simulink model "Led_Switch_Charts"  (R2018b)
settings: Solver=VariableStepAuto  StartTime=0.0  StopTime=10.0  RelTol=1e-3
settings Model: Creator=mostafa  LastModifiedBy=mostafa

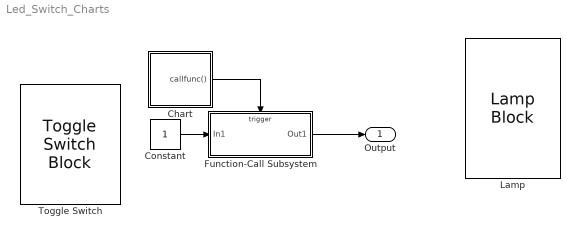
== system Led_Switch_Charts ==
  Chart : Stateflow chart  TreatAsAtomicUnit=on
  Constant : Constant
  Function-Call Subsystem : Subsystem  TreatAsAtomicUnit=on
  Lamp : LampBlock  WebBlockId=14
  Toggle Switch : ToggleSwitchBlock  WebBlockId=11
      settings: Values={{'Off', 'On'}, [0 1]}
  "Output " : Outport
  wires:
  Function-Call Subsystem/1(Out1) -> "Output "/1
  Chart/1(callfunc()) -> Function-Call Subsystem/Trigger
  Constant/1 -> Function-Call Subsystem/1(In1)

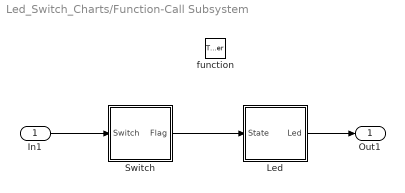
== system Led_Switch_Charts/Function-Call Subsystem ==
  In1 : Inport
  function : TriggerPort  TriggerType=function-call  VariantControl=Variant
  Led : Stateflow chart  TreatAsAtomicUnit=on
  Switch : Stateflow chart  TreatAsAtomicUnit=on
  Out1 : Outport
  wires:
  In1/1 -> Switch/1(Switch)
  Switch/1(Flag) -> Led/1(State)
  Led/1(Led) -> Out1/1

== stateflow chart Led_Switch_Charts/Function-Call Subsystem/Led ==
  (default) -> (junction 18) : % Toggle Led
  (junction 18) -> (junction 19) [order 1] : [State == 1]
  (junction 18) -> (junction 20) [order 2] : {Led = 0;}
  (junction 19) -> (junction 21) : {Led = 1;}
  (junction 21) -> (junction 20)
  (junction 20) -> (junction 22)
  data: Led output; State input

== stateflow chart Led_Switch_Charts/Chart ==
  state CallFunction
    en:
    du:
    ex:
  (default) -> CallFunction
  CallFunction -> CallFunction : [after(5,msec)]{callfunc;}
  events: callfunc output FUNCTION_CALL_EVENT

== stateflow chart Led_Switch_Charts/Function-Call Subsystem/Switch ==
  (default) -> (junction 7) : % Check Button
  (junction 7) -> (junction 8) [order 1] : [Switch == 1]
  (junction 7) -> (junction 9) [order 2] : {Flag = 0;}
  (junction 8) -> (junction 10) : {Flag = 1;}
  (junction 10) -> (junction 9)
  (junction 9) -> (junction 11)
  data: Switch input; Flag output
